simulink model "ans1_65070121_155_168"  (R2024b)
settings: Solver=FixedStepAuto  StartTime=0.0  StopTime=10  FixedStep=0.001  RelTol=1e-3
settings Model: Creator=picha  LastModifiedBy=picha

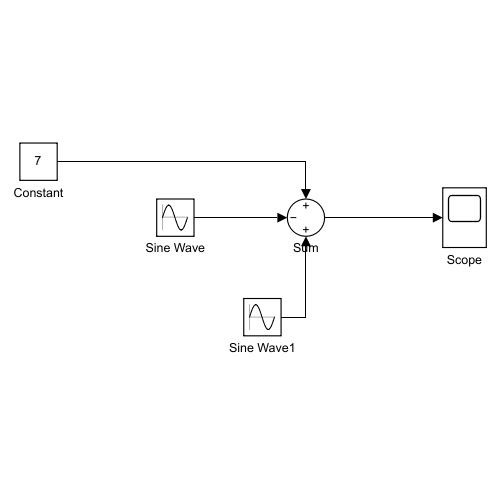
[thumbnail: Simulink's stored preview of the top-level diagram]
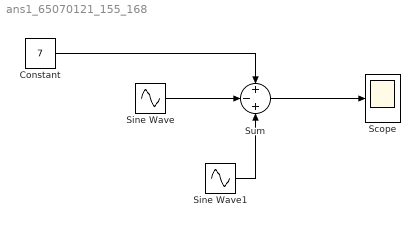
== system ans1_65070121_155_168 ==
  Constant : Constant  Value=7
  Scope : Scope
  Sine Wave : Sin  Amplitude=10  Frequency=40  Phase=pi/6  SampleTime=0
  Sine Wave1 : Sin  Amplitude=4  Frequency=60  SampleTime=0
  Sum : Sum  Inputs=+-+
  wires:
  Constant/1 -> Sum/1
  Sine Wave/1 -> Sum/2
  Sine Wave1/1 -> Sum/3
  Sum/1 -> Scope/1
